simulink model "intelligent_vehicle_example1"  (R2017a)
settings: Solver=VariableStepAuto  StartTime=0.0  StopTime=10.0  RelTol=1e-3
model workspace (MAT data in the model file):
  a = 1
  b = 2
  c = 3
  d = 4
libraries: simulink x1
settings Model: Creator=edward  LastModifiedBy=edward

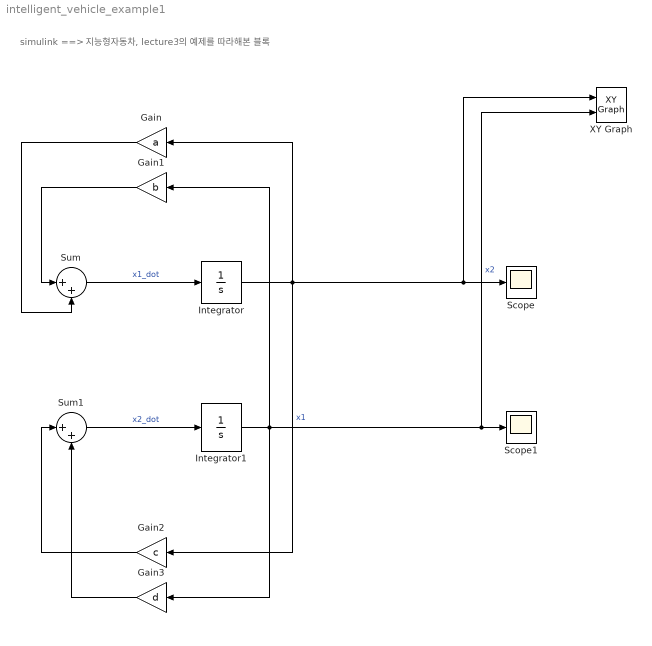
== system intelligent_vehicle_example1 ==
  note: simulink ==> 지능형자동차, lecture3의 예제를 따라해본 블록
  Gain : Gain  Gain=a
  Gain1 : Gain  Gain=b
  Gain2 : Gain  Gain=c
  Gain3 : Gain  Gain=d
  Integrator : Integrator  InitialCondition=-0.1
  Integrator1 : Integrator
  Scope : Scope
  Scope1 : Scope
  Sum : Sum  Inputs=|++
  Sum1 : Sum  Inputs=|++
  XY Graph : simulink/Sinks/XY Graph  xmin=-1  xmax=1  ymin=-1  ymax=1  st=-1
  wires:
  Integrator/1 -> Scope/1, XY Graph/1, Gain2/1, Gain/1  "x1"
  Integrator1/1 -> XY Graph/2, Scope1/1, Gain3/1, Gain1/1  "x2"
  Sum1/1 -> Integrator1/1  "x2_dot"
  Gain2/1 -> Sum1/1
  Sum/1 -> Integrator/1  "x1_dot"
  Gain3/1 -> Sum1/2
  Gain/1 -> Sum/2
  Gain1/1 -> Sum/1
